simulink model "vehicle_hostmodel_2022b_Vignesh"  (R2022b)
settings: Solver=VariableStepAuto  StartTime=0  StopTime=1000  RelTol=1e-3
model workspace (MAT data in the model file):
  finalint = 0
  firstWarning = 1
  originalScenarioChecksum = '114339432DE22364D47BB28FC96DC10C'
undefined symbols (not defined in the file): Acceleration, ActorID, AngularVelocity, cameraParams, curvature, DefaultGear, DEND_B, DEND_S, DEND_T, direction, DiscIntNeverNeededParam, driving, gradbp, L, LF, LR, m, matlabshared, MAX_BRAKE, MAX_STEER, MAX_TORQUE, MCAR, MIN_BRAKE, MIN_STEER, MIN_TORQUE, n, NUMD_B, NUMD_S, NUMD_T, Pitch, Pose, Position, psi_o, R, Roll, RRdamp, SceneInfo, sigbuilder_block, STEER_RATIO, stopSign_ID, Tdead, thetaRefs, TL_ID, trackingParams, TrackWidth, Ts, ts, Vdead, Velocity, WB, X_o, xRef2s, Y_o, Yaw, yRef2, yRef2s
libraries: drivingscenarioandsensors x11, simulink x10, roadrunnerscenario x9, slrealtimeutilitieslib x7, slrealtimeiplib x7, simulink_extras x5, drivingvehiclecontroller x3, trackingutilitieslib x3, robotalgslib x2, slpidlib x2, drivinglib x2, eeGeneralControl x1
(part 5 of 5)

== stateflow chart vehicle_hostmodel_2022b_Vignesh/Behavioural Planner2/Chart ==
  settings: updateMethod=DISCRETE  sampleTime=Ts
  state Stationary
    du:
    VelCmd = 0;
    CurrentVelCmd = VelCmd;
    Navi = 0;
    Trans = 0;
    StopSim = 0;
  state Navigation
    state RailCrossing
      state Approaching
        en:
        ACC = 1;
        Tgap = 0;
        Trans = 0;
      state Stop
        en:
        VelCmd = 0;
        ACC = 0;
        CurrentVelCmd = VelCmd;
      state ExitScene
        en:
        ExitFlag = 1;
      state Transition
        en:
        Tgap = 1;
        Trans = 1;
        VelCmd = SceneSpeed;
        CurrentVelCmd = VelCmd;
      (default) -> Navigation.RailCrossing.Approaching
      Navigation.RailCrossing.Approaching -> Navigation.RailCrossing.Stop [order 1] : [D2S <= 4]
      Navigation.RailCrossing.Stop -> Navigation.RailCrossing.Transition : [RRCross == 0]
      Navigation.RailCrossing.Approaching -> Navigation.RailCrossing.ExitScene [order 2] : [SceneID ~= 10]
      Navigation.RailCrossing.Transition -> Navigation.RailCrossing.ExitScene : [SceneID == 0]
    state RoundAbout
      state Approaching
        en:
        ACC = 1;
        Trans = 0;
        Tgap = 0;
      state Stop
        en:
        VelCmd = 0;
        ACC = 0;
        CurrentVelCmd = VelCmd;
      state ExitScene
        en:
        ExitFlag = 1;
      state Transition
        en:
        Tgap = 1;
        Trans = 1;
        VelCmd = SceneSpeed;
        CurrentVelCmd = VelCmd;
      (default) -> Navigation.RoundAbout.Approaching
      Navigation.RoundAbout.Approaching -> Navigation.RoundAbout.Stop [order 1] : [D2S <= 4]
      Navigation.RoundAbout.Stop -> Navigation.RoundAbout.Transition : [Clear2Go == 1]
      Navigation.RoundAbout.Approaching -> Navigation.RoundAbout.ExitScene [order 2] : [SceneID ~= 9]
      Navigation.RoundAbout.Transition -> Navigation.RoundAbout.ExitScene : [SceneID == 0]
    state DestCheck
      en,du:
      % dest reached?
      (default) -> (junction 47)
      (junction 47) -> (junction 48) [order 1] : [D2D < 2]
      (junction 48) -> (junction 50) : {DestReached = 1;}
      (junction 47) -> (junction 49) [order 2] : {DestReached = 0;}
      (junction 50) -> (junction 49) : {StopSim = 1;}
      (junction 49) -> (junction 51)
    state TrafficLight
      state Stop
        en:
        %CurrentVelCmd = VelCmd;
        %du:
        %if D2S < 7
        % VelCmd = 0;
        %end
      state Approaching
        en:
        Tgap = 0;
        Trans = 0;
        %if TLstate(1,4) == 1
        ACC = 1;
        %else
        % ACC = 0;
        %end
      state Transition
        en:
        Trans = 1;
        ACC = 0;
        Tgap = 1;
        VelCmd = SceneSpeed;
        CurrentVelCmd = VelCmd;
      state ExitScene
        en:
        ExitFlag = 1;
      (default) -> Navigation.TrafficLight.Approaching
      Navigation.TrafficLight.Approaching -> Navigation.TrafficLight.Stop [order 1] : [D2S <= 4]
      Navigation.TrafficLight.Transition -> Navigation.TrafficLight.Approaching [order 2] : [TLstate(1,4) == 1]
      Navigation.TrafficLight.Stop -> Navigation.TrafficLight.Transition : [TLstate(1,4) == 3]
      Navigation.TrafficLight.Approaching -> Navigation.TrafficLight.Transition [order 2] : [TLstate(1,4) == 3]
      Navigation.TrafficLight.Approaching -> Navigation.TrafficLight.ExitScene [order 3] : [SceneID ~= 8]
      Navigation.TrafficLight.Transition -> Navigation.TrafficLight.ExitScene [order 1] : [SceneID == 0]
    state SceneRecognition
      en :
      VelCmd = RoadSpeed;
      CurrentVelCmd = VelCmd;
      ExitFlag = 0;
    state Go
      en:
      VelCmd = RoadSpeed;
      CurrentVelCmd = VelCmd;
      Trans = 0;
      ExitFlag = 0;
      ACC = 0;
    state StopSign
      state Approaching
        en:
        ACC = 1;
        Trans = 0;
        Tgap = 0;
      state Stop
        en:
        VelCmd = 0;
        ACC = 0;
        CurrentVelCmd = VelCmd;
      state ExitScene
        en:
        ExitFlag = 1;
      state Transition
        en:
        Trans = 1;
        ACC = 0;
        Tgap = 1;
        VelCmd = SceneSpeed;
        CurrentVelCmd = VelCmd;
      (default) -> Navigation.StopSign.Approaching
      Navigation.StopSign.Approaching -> Navigation.StopSign.Stop [order 1] : [D2S <= 7]
      Navigation.StopSign.Stop -> Navigation.StopSign.Transition : [after(3,sec) && Clear2Go == 1]
      Navigation.StopSign.Approaching -> Navigation.StopSign.ExitScene [order 2] : [SceneID ~= 7]
      Navigation.StopSign.Transition -> Navigation.StopSign.ExitScene : [SceneID == 0]
    Go -> RailCrossing [order 2] : [SceneID == 10]
    SceneRecognition -> RailCrossing [order 1] : [SceneID == 10]
    RailCrossing -> Go : [ExitFlag == 1]
    Go -> RoundAbout [order 4] : [SceneID == 9]
    SceneRecognition -> RoundAbout [order 2] : [SceneID == 9]
    RoundAbout -> Go : [ExitFlag == 1]
    (default) -> DestCheck
    SceneRecognition -> TrafficLight [order 4] : [SceneID == 8]
    DestCheck -> SceneRecognition : [DestReached == 0]
    Go -> TrafficLight [order 3] : [SceneID == 8]
    SceneRecognition -> DestCheck [order 5] : [D2D < 2]
    SceneRecognition -> StopSign [order 3] : [SceneID == 7]
    TrafficLight -> Go : [ExitFlag == 1]
    StopSign -> Go : [ExitFlag == 1]
    Go -> DestCheck [order 1] : [SceneID == 0]
    Go -> StopSign [order 5] : [SceneID == 7]
  (default) -> Stationary
  Stationary -> Navigation : [Navigate == 1]
  Navigation -> Stationary : [Navigate == 0 || DestReached == 1]
  data: TLstate input; ApproachingSpeed input; ObjectDist input; SceneSpeed input; SDist input; RRCross input; D2S input; DestReached local; Navigate input; ExitFlag local; D2D input; Clear2Go input; RoadSpeed input; CurrentVelCmd local; Navi local; VelCmd output; SceneID input; ACC output; Tgap output; Trans output; StopSim output

== stateflow chart vehicle_hostmodel_2022b_Vignesh/Behavioural Planner2/Collision Avoidance ==
  state Start
    en:
    Stuck = 0;
    ACC = 0;
    LaneChangeCmd = 0;
    %VelCmd = CurrentVelCmd;
  state Follow
    en:
    ACC = 1;
  state LaneChange
    en:
    LaneChangeCmd = 1;
    ACC=0;
  LaneChange -> Start : [LaneChanged == 1]
  (default) -> Start
  Follow -> LaneChange [order 2] : [LC_ACC == 1]
  Start -> Follow : [ObjAhead == 1]
  Follow -> Start [order 3] : [ObjAhead == 0]
  Follow -> Follow [order 1] : [(EgoSpeed <= MinSpeed) && after(WaitTime,sec)]{Stuck = 1;}
  data: Stuck local; ACC output; WaitTime input; ObjAhead input; MinSpeed input; LaneAvailable input; EgoSpeed input; LC_ACC input; LaneChanged input; LaneChangeCmd output

== stateflow chart vehicle_hostmodel_2022b_Vignesh/Behavioural Planner2/Emergency Stop ==
  state EmergencyCheck
    en:
    EStop = 0;
  state Pullover
    en:
    EStop=1;
  state Stop
    en:
    EStop=2;
  Pullover -> EmergencyCheck : [TechFailure == 0]
  (default) -> EmergencyCheck
  EmergencyCheck -> Pullover [order 1] : [TechFailure == 1]
  EmergencyCheck -> Stop [order 2] : [D2O<=1]
  Stop -> EmergencyCheck : [D2O > 2]
  data: D2O input; TechFailure input; EStop output

== matlab function vehicle_hostmodel_2022b_Vignesh/Behavioural Planner2/MATLAB Function ==
  data: Dest input; D2D output; CurrentPose input
function D2D = fcn(Dest, CurrentPose)
CurrentPose(2) = CurrentPose(2);    %Change sign to negative if flipping signs in tlstart ref pose.
D2D = norm(Dest - CurrentPose(1:2));

== stateflow chart vehicle_hostmodel_2022b_Vignesh/Behavioural Planner2/Routing ==
  state InitialRoute
    en:
    NewRoute = 0;
  state Rerouting
    en:
    NewRoute = 1;
  (default) -> InitialRoute
  InitialRoute -> Rerouting : [ReRoute == 1]
  Rerouting -> InitialRoute : [ReRoute == 0]
  data: ReRoute input; NewRoute output
